simulink model "AdmittanceScanPRBS"  (R2025a)
settings: Solver=VariableStepAuto  StartTime=0.0  StopTime=Tsim  RelTol=1e-3
PreLoadFcn:
  | SimulationTime = 10;
  | AdmittanceScanParameters;
undefined symbols (not defined in the file): Array, Base, BatteryInverter, DiscIntNeverNeededParam, ee_sli_rtmsupport, feeder, fRT, frt, gcbh, GFLBatteryController, GFMBatteryController, gGFM, grid, Grid, line, loadpq, loadstep1, loadstep2, lvrt, LVRT, mGFM, Panel, pll, pmsm, PVController, PVInverter, PVTransformer, scan, time, Ts, VSMbase, windController, windTurbine
libraries: ee_lib x19, eeGeneralControl x17, nesl_utility x16, fl_lib x10, eeTransforms x9, simulink x8, slpidlib x2, batteryecm_lib x1, simulink_extras x1, eePowerMeasurement x1
(part 2 of 4)

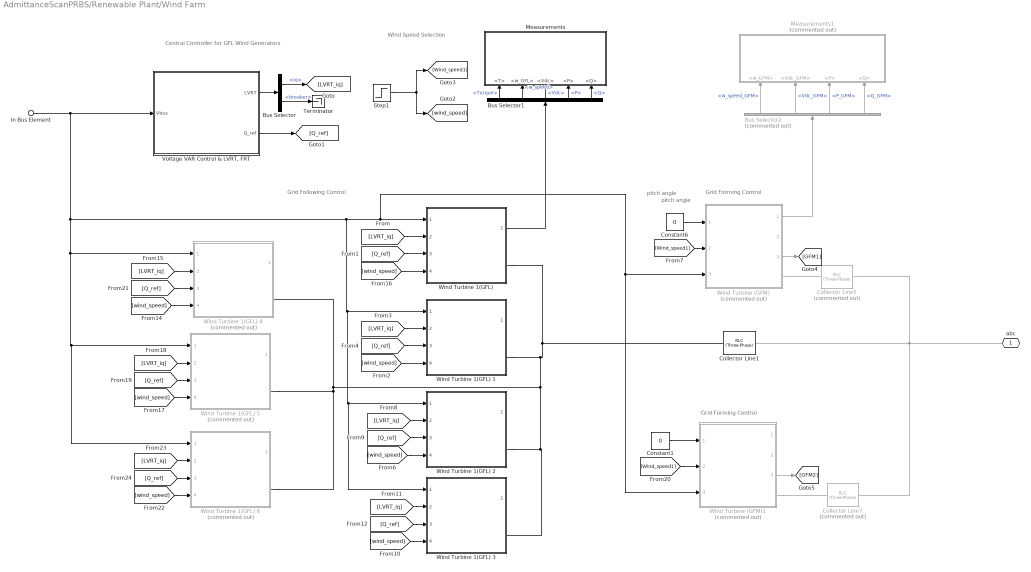
== system AdmittanceScanPRBS/Renewable Plant/Wind Farm ==
  note: Central Controller for GFL Wind Generators
  note: Wind Speed Selection
  note: pitch angle
  note: Grid Following Control
  note: Grid Forming Control
  note: Grid Forming Control
  note: pitch angle
  In Bus Element : Inport  PortName=Vbus
  Bus Selector : BusSelector  OutputSignals=iq,breaker
  Bus Selector1 : BusSelector  OutputSignals=Torque,w_speed,Vdc,P,Q
  Bus Selector2 : BusSelector  Commented=on  OutputSignals=w_speed_GFM,Vdc_GFM,P_GFM,Q_GFM
  Collector Line1 : ee_lib/Passive/RLC Assemblies/RLC (Three-Phase)  port_option=ee.enum.threePhasePort.composite  component_structure=ee.enum.rlc.structure.SeriesRL  R=feeder.r*0.002 Ohm  L=feeder.l*0.002 H  C=1e-6 F  R_parasitic=0 Ohm  G_parasitic=0 1/Ohm  IL_specify=off  IL_priority=High  IL=[0, 0, 0] A  IL_nominal_specify=off  IL_nominal_value=1  IL_nominal_unit=A  VC_specify=off  VC_priority=High  VC=[0, 0, 0] V  VC_nominal_specify=off  VC_nominal_value=1  VC_nominal_unit=V
      settings: InternalSimscapePortConfiguration="{\"Bottom\":[],\"Left\":[{\"id\":\"N1\",\"label\":\"~1\",\"type\":\"foundation.electrical.three_phase\"}],\"Right\":[{\"id\":\"N2\",\"label\":\"~2\",\"type\":\"foundation.electrical.three_phase\"}],\"Top\":[]}"
  Collector Line5 : ee_lib/Passive/RLC Assemblies/RLC (Three-Phase)  Commented=on  port_option=ee.enum.threePhasePort.composite  component_structure=ee.enum.rlc.structure.SeriesRL  R=feeder.r*0.005 Ohm  L=feeder.l*0.005 H  C=1e-6 F  R_parasitic=0 Ohm  G_parasitic=0 1/Ohm  IL_specify=off  IL_priority=High  IL=[0, 0, 0] A  IL_nominal_specify=off  IL_nominal_value=1  IL_nominal_unit=A  VC_specify=off  VC_priority=High  VC=[0, 0, 0] V  VC_nominal_specify=off  VC_nominal_value=1  VC_nominal_unit=V
      settings: InternalSimscapePortConfiguration="{\"Bottom\":[],\"Left\":[{\"id\":\"N1\",\"label\":\"~1\",\"type\":\"foundation.electrical.three_phase\"}],\"Right\":[{\"id\":\"N2\",\"label\":\"~2\",\"type\":\"foundation.electrical.three_phase\"}],\"Top\":[]}"
  Collector Line7 : ee_lib/Passive/RLC Assemblies/RLC (Three-Phase)  Commented=on  port_option=ee.enum.threePhasePort.composite  component_structure=ee.enum.rlc.structure.SeriesRL  R=feeder.r*0.001 Ohm  L=feeder.l*0.001 H  C=1e-6 F  R_parasitic=0 Ohm  G_parasitic=0 1/Ohm  IL_specify=off  IL_priority=High  IL=[0, 0, 0] A  IL_nominal_specify=off  IL_nominal_value=1  IL_nominal_unit=A  VC_specify=off  VC_priority=High  VC=[0, 0, 0] V  VC_nominal_specify=off  VC_nominal_value=1  VC_nominal_unit=V
      settings: InternalSimscapePortConfiguration="{\"Bottom\":[],\"Left\":[{\"id\":\"N1\",\"label\":\"~1\",\"type\":\"foundation.electrical.three_phase\"}],\"Right\":[{\"id\":\"N2\",\"label\":\"~2\",\"type\":\"foundation.electrical.three_phase\"}],\"Top\":[]}"
  Constant1 : Constant  Value=0
  Constant6 : Constant  Value=0
  Measurements : Subsystem
  Measurements1 : Subsystem  Commented=on
  Step1 : Step  Time=time.renewablevariation  Before=12  After=10.5  SampleTime=Ts  ZeroCross=off
  Terminator : Terminator
  "Voltage VAR Control & LVRT, FRT" : Subsystem
      mask Display: image('$imagefile'); % Use "Edit Image" on toolstrip to change.
  Wind Turbine (GFM) : Subsystem  Commented=on  ReferencedSubsystem=gfmWind  Control=VSM Using Turbine Inertia  V_ref=gGFM.vref  Q_ref=gGFM.qref  Kq=gGFM.kq  Kt=gGFM.kt  KqI=mGFM.kq  Kp=mGFM.kp  Kd=gGFM.kd  Kj=gGFM.kj  H=mGFM.h  D=mGFM.d  Vd_ref=mGFM.Vd  frequency1=gGFM.fref  frequency=mGFM.fref  x_vir=mGFM.x_vir  x_vir1=gGFM.r_vir  r_vir1=gGFM.x_vir  Imax1=gGFM.Imax  Imax=mGFM.Imax  r_vir=mGFM.r_vir  Kpq_mpp=pmsm.lq*pmsm.alpha  Kpd_mpp=pmsm.ld*pmsm.alpha  Kiq_mpp=pmsm.rs*pmsm.alpha  Kid_mpp=pmsm.rs*pmsm.alpha  Kpq=pmsm.lq*pmsm.alpha  Kpd=pmsm.ld*pmsm.alpha  Kiq=pmsm.rs*pmsm.alpha  Kid=pmsm.rs*pmsm.alpha  Kp_dc_sm=mGFM.kpdc  Ki_dc_sm=mGFM.kidc  wt1=0.01  rt1=0.01  pitch1=windTurbine.pitch  cp1=windTurbine.cp  airDensity1=windTurbine.airDensity  TSR1=windTurbine.TSR  Radius1=windTurbine.turbineRadius  wt=0.01  rt=0.01  pitch=windTurbine.pitch  cp=windTurbine.cp  airDensity=windTurbine.airDensity  Radius=windTurbine.turbineRadius  TSR=windTurbine.TSR  Inertia1=windTurbine.inertia  Inertia=windTurbine.inertia  psim1=pmsm.psim  p1=pmsm.p  Rs1=pmsm.rs  Lq1=pmsm.lq  Ld1=pmsm.ld  Ld=pmsm.ld  Lq=pmsm.lq  Rs=pmsm.rs  p=pmsm.p  psim=pmsm.psim
  Wind Turbine (GFM)1 : Subsystem  Commented=on  ReferencedSubsystem=gfmWind  Control=VSM Using Turbine Inertia  V_ref=gGFM.vref  Q_ref=gGFM.qref  Kq=gGFM.kq  Kt=gGFM.kt  KqI=mGFM.kq  Kp=mGFM.kp  Kd=gGFM.kd  Kj=gGFM.kj  H=mGFM.h  D=mGFM.d  Vd_ref=mGFM.Vd  frequency1=gGFM.fref  frequency=mGFM.fref  x_vir=mGFM.x_vir  x_vir1=gGFM.r_vir  r_vir1=gGFM.x_vir  Imax1=gGFM.Imax  Imax=mGFM.Imax  r_vir=mGFM.r_vir  Kpq_mpp=pmsm.lq*pmsm.alpha  Kpd_mpp=pmsm.ld*pmsm.alpha  Kiq_mpp=pmsm.rs*pmsm.alpha  Kid_mpp=pmsm.rs*pmsm.alpha  Kpq=pmsm.lq*pmsm.alpha  Kpd=pmsm.ld*pmsm.alpha  Kiq=pmsm.rs*pmsm.alpha  Kid=pmsm.rs*pmsm.alpha  Kp_dc_sm=mGFM.kpdc  Ki_dc_sm=mGFM.kidc  wt1=0.01  rt1=0.01  pitch1=windTurbine.pitch  cp1=windTurbine.cp  airDensity1=windTurbine.airDensity  TSR1=windTurbine.TSR  Radius1=windTurbine.turbineRadius  wt=0.01  rt=0.01  pitch=windTurbine.pitch  cp=windTurbine.cp  airDensity=windTurbine.airDensity  Radius=windTurbine.turbineRadius  TSR=windTurbine.TSR  Inertia1=windTurbine.inertia  Inertia=windTurbine.inertia  psim1=pmsm.psim  p1=pmsm.p  Rs1=pmsm.rs  Lq1=pmsm.lq  Ld1=pmsm.ld  Ld=pmsm.ld  Lq=pmsm.lq  Rs=pmsm.rs  p=pmsm.p  psim=pmsm.psim
  Wind Turbine 1(GFL) : Subsystem  ReferencedSubsystem=WindGFLMpp  p=pmsm.p  psim=pmsm.psim  Rs=pmsm.rs  Ld=pmsm.ld  Lq=pmsm.lq  Kdip_sm=pmsm.ld*pmsm.alpha  Kdii_sm=pmsm.rs*pmsm.alpha  Kqip_sm=pmsm.lq*pmsm.alpha  Kqii_sm=pmsm.rs*pmsm.alpha  airDensity=windTurbine.airDensity  turbineRadius=windTurbine.turbineRadius  pitch=windTurbine.pitch  TSR=windTurbine.TSR  cp=windTurbine.cp  wt=0.01  rt=0.01  Inertia=windTurbine.inertia  Kp_dc=windController.kpv  Ki_dc=windController.kiv  Kdpi_g=windController.kpic  Kdii_g=windController.kiic  Kqpi_g=windController.kpic  Kqii_g=windController.kiic
  Wind Turbine 1(GFL) 1 : Subsystem  ReferencedSubsystem=WindGFLMpp  p=pmsm.p  psim=pmsm.psim  Rs=pmsm.rs  Ld=pmsm.ld  Lq=pmsm.lq  Kdip_sm=pmsm.ld*pmsm.alpha  Kdii_sm=pmsm.rs*pmsm.alpha  Kqip_sm=pmsm.lq*pmsm.alpha  Kqii_sm=pmsm.rs*pmsm.alpha  airDensity=windTurbine.airDensity  turbineRadius=windTurbine.turbineRadius  pitch=windTurbine.pitch  TSR=windTurbine.TSR  cp=windTurbine.cp  wt=0.01  rt=0.01  Inertia=windTurbine.inertia  Kp_dc=windController.kpv  Ki_dc=windController.kiv  Kdpi_g=windController.kpic  Kdii_g=windController.kiic  Kqpi_g=windController.kpic  Kqii_g=windController.kiic
  Wind Turbine 1(GFL) 2 : Subsystem  ReferencedSubsystem=WindGFLMpp  p=pmsm.p  psim=pmsm.psim  Rs=pmsm.rs  Ld=pmsm.ld  Lq=pmsm.lq  Kdip_sm=pmsm.ld*pmsm.alpha  Kdii_sm=pmsm.rs*pmsm.alpha  Kqip_sm=pmsm.lq*pmsm.alpha  Kqii_sm=pmsm.rs*pmsm.alpha  airDensity=windTurbine.airDensity  turbineRadius=windTurbine.turbineRadius  pitch=windTurbine.pitch  TSR=windTurbine.TSR  cp=windTurbine.cp  wt=0.01  rt=0.01  Inertia=windTurbine.inertia  Kp_dc=windController.kpv  Ki_dc=windController.kiv  Kdpi_g=windController.kpic  Kdii_g=windController.kiic  Kqpi_g=windController.kpic  Kqii_g=windController.kiic
  Wind Turbine 1(GFL) 3 : Subsystem  ReferencedSubsystem=WindGFLMpp  p=pmsm.p  psim=pmsm.psim  Rs=pmsm.rs  Ld=pmsm.ld  Lq=pmsm.lq  Kdip_sm=pmsm.ld*pmsm.alpha  Kdii_sm=pmsm.rs*pmsm.alpha  Kqip_sm=pmsm.lq*pmsm.alpha  Kqii_sm=pmsm.rs*pmsm.alpha  airDensity=windTurbine.airDensity  turbineRadius=windTurbine.turbineRadius  pitch=windTurbine.pitch  TSR=windTurbine.TSR  cp=windTurbine.cp  wt=0.01  rt=0.01  Inertia=windTurbine.inertia  Kp_dc=windController.kpv  Ki_dc=windController.kiv  Kdpi_g=windController.kpic  Kdii_g=windController.kiic  Kqpi_g=windController.kpic  Kqii_g=windController.kiic
  Wind Turbine 1(GFL) 4 : Subsystem  Commented=on  ReferencedSubsystem=WindGFLMpp  p=pmsm.p  psim=pmsm.psim  Rs=pmsm.rs  Ld=pmsm.ld  Lq=pmsm.lq  Kdip_sm=pmsm.ld*pmsm.alpha  Kdii_sm=pmsm.rs*pmsm.alpha  Kqip_sm=pmsm.lq*pmsm.alpha  Kqii_sm=pmsm.rs*pmsm.alpha  airDensity=windTurbine.airDensity  turbineRadius=windTurbine.turbineRadius  pitch=windTurbine.pitch  TSR=windTurbine.TSR  cp=windTurbine.cp  wt=0.01  rt=0.01  Inertia=windTurbine.inertia  Kp_dc=windController.kpv  Ki_dc=windController.kiv  Kdpi_g=windController.kpic  Kdii_g=windController.kiic  Kqpi_g=windController.kpic  Kqii_g=windController.kiic
  Wind Turbine 1(GFL) 5 : Subsystem  Commented=on  ReferencedSubsystem=WindGFLMpp  p=pmsm.p  psim=pmsm.psim  Rs=pmsm.rs  Ld=pmsm.ld  Lq=pmsm.lq  Kdip_sm=pmsm.ld*pmsm.alpha  Kdii_sm=pmsm.rs*pmsm.alpha  Kqip_sm=pmsm.lq*pmsm.alpha  Kqii_sm=pmsm.rs*pmsm.alpha  airDensity=windTurbine.airDensity  turbineRadius=windTurbine.turbineRadius  pitch=windTurbine.pitch  TSR=windTurbine.TSR  cp=windTurbine.cp  wt=0.01  rt=0.01  Inertia=windTurbine.inertia  Kp_dc=windController.kpv  Ki_dc=windController.kiv  Kdpi_g=windController.kpic  Kdii_g=windController.kiic  Kqpi_g=windController.kpic  Kqii_g=windController.kiic
  Wind Turbine 1(GFL) 6 : Subsystem  Commented=on  ReferencedSubsystem=WindGFLMpp  p=pmsm.p  psim=pmsm.psim  Rs=pmsm.rs  Ld=pmsm.ld  Lq=pmsm.lq  Kdip_sm=pmsm.ld*pmsm.alpha  Kdii_sm=pmsm.rs*pmsm.alpha  Kqip_sm=pmsm.lq*pmsm.alpha  Kqii_sm=pmsm.rs*pmsm.alpha  airDensity=windTurbine.airDensity  turbineRadius=windTurbine.turbineRadius  pitch=windTurbine.pitch  TSR=windTurbine.TSR  cp=windTurbine.cp  wt=0.01  rt=0.01  Inertia=windTurbine.inertia  Kp_dc=windController.kpv  Ki_dc=windController.kiv  Kdpi_g=windController.kpic  Kdii_g=windController.kiic  Kqpi_g=windController.kpic  Kqii_g=windController.kiic
  abc : PMIOPort  Side=Right
  wires:
  "Voltage VAR Control & LVRT, FRT"/1(LVRT) -> Bus Selector/1
  Bus Selector/2 -> Terminator/1  "<breaker>"
  Bus Selector1/4 -> Measurements/4(<P>)  "<P>"
  Bus Selector1/5 -> Measurements/5(<Q>)  "<Q>"
  Bus Selector1/1 -> Measurements/1(<T>)  "<Torque>"
  Bus Selector1/3 -> Measurements/3(<Vdc>)  "<Vdc>"
  Bus Selector1/2 -> Measurements/2(<w_GFL>)  "<w_speed>"
  "Voltage VAR Control & LVRT, FRT"/2(Q_ref) -> [Q_ref]
  Bus Selector/1 -> [LVRT_iq]  "<iq>"
  Wind Turbine 1(GFL)/1 -> Bus Selector1/1
  Wind Turbine (GFM)/3 -> [GFM1]
  Bus Selector2/4 -> Measurements1/4(<Q>)  "<Q_GFM>"
  Bus Selector2/3 -> Measurements1/3(<P>)  "<P_GFM>"
  Bus Selector2/1 -> Measurements1/1(<w_GFM>)  "<w_speed_GFM>"
  Bus Selector2/2 -> Measurements1/2(<Vdc_GFM>)  "<Vdc_GFM>"
  Wind Turbine (GFM)/1 -> Bus Selector2/1
  Step1/1 -> [Wind_speed1], [wind_speed]
  [LVRT_iq] -> Wind Turbine 1(GFL) 4/2
  [Q_ref] -> Wind Turbine 1(GFL) 4/3
  [wind_speed] -> Wind Turbine 1(GFL) 4/4
  [LVRT_iq] -> Wind Turbine 1(GFL) 5/2
  [Q_ref] -> Wind Turbine 1(GFL) 5/3
  [wind_speed] -> Wind Turbine 1(GFL) 5/4
  [LVRT_iq] -> Wind Turbine 1(GFL) 6/2
  [Q_ref] -> Wind Turbine 1(GFL) 6/3
  [wind_speed] -> Wind Turbine 1(GFL) 6/4
  [LVRT_iq] -> Wind Turbine 1(GFL)/2
  [Q_ref] -> Wind Turbine 1(GFL)/3
  [wind_speed] -> Wind Turbine 1(GFL)/4
  [LVRT_iq] -> Wind Turbine 1(GFL) 1/2
  [Q_ref] -> Wind Turbine 1(GFL) 1/3
  [wind_speed] -> Wind Turbine 1(GFL) 1/4
  [LVRT_iq] -> Wind Turbine 1(GFL) 2/2
  [Q_ref] -> Wind Turbine 1(GFL) 2/3
  [wind_speed] -> Wind Turbine 1(GFL) 2/4
  [LVRT_iq] -> Wind Turbine 1(GFL) 3/2
  [Q_ref] -> Wind Turbine 1(GFL) 3/3
  [wind_speed] -> Wind Turbine 1(GFL) 3/4
  Constant6/1 -> Wind Turbine (GFM)/1
  [Wind_speed1] -> Wind Turbine (GFM)/2
  Constant1/1 -> Wind Turbine (GFM)1/1
  [Wind_speed1] -> Wind Turbine (GFM)1/2
  Wind Turbine (GFM)1/3 -> [GFM2]
  In Bus Element/1 -> Wind Turbine 1(GFL) 3/1, Wind Turbine 1(GFL) 2/1, Wind Turbine 1(GFL) 1/1, Wind Turbine (GFM)1/3, Wind Turbine (GFM)/3, Wind Turbine 1(GFL)/1, Wind Turbine 1(GFL) 6/1, Wind Turbine 1(GFL) 5/1, Wind Turbine 1(GFL) 4/1, "Voltage VAR Control & LVRT, FRT"/1(Vbus)
  connections:
  Wind Turbine (GFM)/RConn1 -- Collector Line5/LConn1
  Wind Turbine (GFM)1/RConn1 -- Collector Line7/LConn1
  Wind Turbine 1(GFL) 4/RConn1 -- Wind Turbine 1(GFL) 6/RConn1 -- Wind Turbine 1(GFL) 5/RConn1 -- Wind Turbine 1(GFL) 3/RConn1 -- Wind Turbine 1(GFL) 2/RConn1 -- Wind Turbine 1(GFL) 1/RConn1 -- Collector Line1/LConn1 -- Wind Turbine 1(GFL)/RConn1
  Collector Line7/RConn1 -- Collector Line1/RConn1 -- Collector Line5/RConn1 -- abc/RConn1

== system AdmittanceScanPRBS/PLL & Measurements/PLL/Sinusoidal Measurement (PLL, Three-Phase)1 ==
  note: Loop Filter (LF)
  note: Voltage-controlled oscillator (VCO)
  abc : Inport  PortDimensions=3  SampleTime=Ts
  Angle : Subsystem
  Low-Pass Filter (Discrete or Continuous) : eeGeneralControl/Low-Pass Filter (Discrete or Continuous)  K=1/2/pi  T=1e-3  B=inf  A=-inf  init_option=Specify as parameter  x0=F0  Ts=Ts
      settings: LibrarySourceBlock=|
      | eeSinusoidalMeasurementV2/Sinusoidal Measurement
      | (PLL, Three-Phase)/Low-Pass Filter
      | (Discrete or Continuous)
  Moving Average (Variable Frequency) : eeGeneralControl/Moving Average (Variable Frequency)  VariantControl=Variant1  LabelModeActiveChoice=Discrete  f0=F0  fmin=5  x0=0  BufferSize=8192  Ts=Ts
      settings: LibrarySourceBlock=|
      | eeSinusoidalMeasurementV2/Sinusoidal Measurement
      | (PLL, Three-Phase)/Moving Average
      | (Variable Frequency)
  PI : Subsystem
  Park Transform : eeTransforms/Park Transform  AxisAlignment=Q-axis  PowerInvariant=off
  Pythagorian Sum : Fcn  Expr=sqrt(u(1)^2+u(2)^2)
  Selector2 : Selector  InputPortWidth=3  IndexOptions=Index vector (dialog)  Indices=[2]  OutputSizes=1
  freq : Outport  VectorParamsAs1DForOutWhenUnconnected=off
  angle : Outport  Port=2  VectorParamsAs1DForOutWhenUnconnected=off
  mag : Outport  Port=3  VectorParamsAs1DForOutWhenUnconnected=off
  wires:
  Moving Average (Variable Frequency)/1 -> Selector2/1, Pythagorian Sum/1
  Selector2/1 -> PI/1(u)
  Low-Pass Filter (Discrete or Continuous)/1 -> freq/1, Moving Average (Variable Frequency)/1
  Angle/1(theta) -> angle/1, Park Transform/2
  PI/1(y) -> Angle/1(omega), Low-Pass Filter (Discrete or Continuous)/1
  Park Transform/1 -> Moving Average (Variable Frequency)/2
  Pythagorian Sum/1 -> mag/1
  abc/1 -> Park Transform/1

== system AdmittanceScanPRBS/Renewable Plant/PV Plant/100 MWp PV Park ==
  note: PV Park
  LVRT_iq : Inport
  Q_ref : Inport  Port=2
  "Current and Voltage Sensor " : ee_lib/Sensors & Transducers/Current and Voltage Sensor (Three-Phase)  vMeasurementType=ee.enum.vmeasurement.lg  outputUnit=ee.enum.unit.pu  SRated=Base.MVA_base_new A*V  VRated=Base.KV_base_new V  I_specify=off  I_priority=None  I=[0, 0, 0] A  I_nominal_specify=off  I_nominal_value=1  I_nominal_unit=A  V_specify=off  V_priority=None  V=[0, 0, 0] V  V_nominal_specify=off  V_nominal_value=1  V_nominal_unit=V
      settings: InternalSimscapePortConfiguration="{\"Bottom\":[],\"Left\":[{\"id\":\"N1\",\"label\":\"~1\",\"type\":\"foundation.electrical.three_phase\"}],\"Right\":[{\"id\":\"V_output\",\"label\":\"V\",\"type\":\"output\"},{\"id\":\"I_output\",\"label\":\"I\",\"type\":\"output\"},{\"id\":\"N2\",\"label\":\"~2\",\"type\":\"foundation.electrical.three_phase\"}],\"Top\":[]}"
  PS-Simulink Converter25 : nesl_utility/PS-Simulink Converter  PhysicalDomain=network_engine_domain  SubClassName=ps_output  LeftPortType=input  RightPortType=output  PseudoPeriodic=off  Frequencies=[]  VectorFormat=inherit  Unit=inherit  AffineConversion=off
  PV Inverter A2 : Subsystem
  Step2 : Step  Time=time.renewablevariation  Before=600  After=650  SampleTime=Ts
  PV : PMIOPort  Side=Left
  IPV : Outport
  wires:
  PS-Simulink Converter25/1 -> IPV/1
  Q_ref/1 -> PV Inverter A2/3(Q_ref)
  Step2/1 -> PV Inverter A2/1(Insolation1)
  LVRT_iq/1 -> PV Inverter A2/2(LVRT)
  connections:
  PV/RConn1 -- "Current and Voltage Sensor "/RConn3
  PS-Simulink Converter25/LConn1 -- "Current and Voltage Sensor "/RConn2
  PV Inverter A2/RConn1 -- "Current and Voltage Sensor "/LConn1

== system AdmittanceScanPRBS/Renewable Plant/PV Plant/60 MWhr Battery Energy Storage ==
  In Bus Element : Inport  PortName=Vbus
  LVRT_iq : Inport  Port=2
  Current and Voltage Sensor (Three-Phase)5 : ee_lib/Sensors & Transducers/Current and Voltage Sensor (Three-Phase)  vMeasurementType=ee.enum.vmeasurement.lg  outputUnit=ee.enum.unit.pu  SRated=Base.MVA_base_new A*V  VRated=Base.KV_base_new V  I_specify=off  I_priority=None  I=[0, 0, 0] A  I_nominal_specify=off  I_nominal_value=1  I_nominal_unit=A  V_specify=off  V_priority=None  V=[0, 0, 0] V  V_nominal_specify=off  V_nominal_value=1  V_nominal_unit=V
      settings: InternalSimscapePortConfiguration="{\"Bottom\":[],\"Left\":[{\"id\":\"N1\",\"label\":\"~1\",\"type\":\"foundation.electrical.three_phase\"}],\"Right\":[{\"id\":\"V_output\",\"label\":\"V\",\"type\":\"output\"},{\"id\":\"I_output\",\"label\":\"I\",\"type\":\"output\"},{\"id\":\"N2\",\"label\":\"~2\",\"type\":\"foundation.electrical.three_phase\"}],\"Top\":[]}"
  Inverter and DC-DC Converter : Subsystem
  L Filter : ee_lib/Passive/RLC Assemblies/RLC (Three-Phase)  port_option=ee.enum.threePhasePort.composite  component_structure=ee.enum.rlc.structure.L  R=1e-3 Ohm  L=PVInverter.L H  C=1e-6 F  R_parasitic=0 Ohm  G_parasitic=0 1/Ohm  IL_specify=off  IL_priority=High  IL=[0, 0, 0] A  IL_nominal_specify=off  IL_nominal_value=1  IL_nominal_unit=A  VC_specify=off  VC_priority=High  VC=[0, 0, 0] V  VC_nominal_specify=off  VC_nominal_value=1  VC_nominal_unit=V
      settings: InternalSimscapePortConfiguration="{\"Bottom\":[],\"Left\":[{\"id\":\"N1\",\"label\":\"~1\",\"type\":\"foundation.electrical.three_phase\"}],\"Right\":[{\"id\":\"N2\",\"label\":\"~2\",\"type\":\"foundation.electrical.three_phase\"}],\"Top\":[]}"
  Measurement5 : Subsystem
  PS-Simulink Converter10 : nesl_utility/PS-Simulink Converter  PhysicalDomain=network_engine_domain  SubClassName=ps_output  LeftPortType=input  RightPortType=output  PseudoPeriodic=off  Frequencies=[]  VectorFormat=inherit  Unit=inherit  AffineConversion=off
  PS-Simulink Converter9 : nesl_utility/PS-Simulink Converter  PhysicalDomain=network_engine_domain  SubClassName=ps_output  LeftPortType=input  RightPortType=output  PseudoPeriodic=off  Frequencies=[]  VectorFormat=inherit  Unit=inherit  AffineConversion=off
  Variant Subsystem : Subsystem  Variant=on  VariantControlMode=label  LabelModeActiveChoice=BESSGridSupporting  mask{LabelModeActiveChoice=BESSGridSupporting}
      mask prompts: LabelModeActiveChoice "Choose BESS Controller"
      mask TypeOptions LabelModeActiveChoice: LabelModeActiveChoice
  abc : PMIOPort  Side=Right
  Bat : Outport
  wires:
  In Bus Element/1 -> Variant Subsystem/2(Vbus)
  Variant Subsystem/1(mabc) -> Inverter and DC-DC Converter/1(m_abc)
  PS-Simulink Converter9/1 -> Measurement5/2(u)
  PS-Simulink Converter10/1 -> Measurement5/1(In1)
  Measurement5/2(Bat) -> Bat/1, Variant Subsystem/4(Bat)
  LVRT_iq/1 -> Variant Subsystem/3(LVRT_iq)
  Measurement5/1(ipv1) -> Variant Subsystem/1(ipv2)
  connections:
  abc/RConn1 -- Current and Voltage Sensor (Three-Phase)5/RConn3
  Inverter and DC-DC Converter/RConn1 -- L Filter/LConn1
  Current and Voltage Sensor (Three-Phase)5/LConn1 -- L Filter/RConn1
  Current and Voltage Sensor (Three-Phase)5/RConn1 -- PS-Simulink Converter10/LConn1
  PS-Simulink Converter9/LConn1 -- Current and Voltage Sensor (Three-Phase)5/RConn2

== system AdmittanceScanPRBS/Renewable Plant/PV Plant/PV Plant Controller  ==
  In Bus Element14 : Inport  PortName=Vbus
  Terminator : Terminator
  "Voltage VAR Control & LVRT, FRT" : Subsystem
      mask Display: image('$imagefile'); % Use "Edit Image" on toolstrip to change.
  Q_ref : Outport
  wires:
  In Bus Element14/1 -> "Voltage VAR Control & LVRT, FRT"/1(Vbus)
  "Voltage VAR Control & LVRT, FRT"/2(Q_ref) -> Q_ref/1
  "Voltage VAR Control & LVRT, FRT"/1(LVRT) -> Terminator/1

== system AdmittanceScanPRBS/Renewable Plant/Wind Farm/Measurements ==
  <T> : Inport
  <w_GFL> : Inport  Port=2
  <Vdc> : Inport  Port=3
  <P> : Inport  Port=4
  <Q> : Inport  Port=5
  Terminator{,1..4} (5 alike) : Terminator
  wires:
  <Vdc>/1 -> Terminator2/1  "Vdc_GFL"
  <Q>/1 -> Terminator4/1
  <w_GFL>/1 -> Terminator1/1
  <T>/1 -> Terminator/1
  <P>/1 -> Terminator3/1

== system AdmittanceScanPRBS/Renewable Plant/Wind Farm/Measurements1 ==
  <w_GFM> : Inport
  <Vdc_GFM> : Inport  Port=2
  <P> : Inport  Port=3
  <Q> : Inport  Port=4
  Terminator{1..4} (4 alike) : Terminator
  wires:
  <P>/1 -> Terminator3/1
  <w_GFM>/1 -> Terminator1/1
  <Q>/1 -> Terminator4/1
  <Vdc_GFM>/1 -> Terminator2/1

== system AdmittanceScanPRBS/Renewable Plant/Wind Farm/Voltage VAR Control & LVRT, FRT ==
  In Bus Element : Inport  PortName=Vbus  Element=Vmag
  In Bus Element1 : Inport  PortName=Vbus  Element=w
  Data Type Conversion : DataTypeConversion  RndMeth=Nearest  SaturateOnIntegerOverflow=off
  Delay : Delay  DelayLength=100
  Frequency RideThrough : Subsystem
  LVRT Characterstics : Subsystem
  OR : Logic  Operator=OR  IconShape=distinctive  AllPortsSameDT=off  OutDataTypeStr=boolean
  Unit Delay : UnitDelay  SampleTime=-1  HasFrameUpgradeWarning=on
  V_ref : Constant  Value=windController.vRef  SampleTime=Ts
  Voltage Control : Subsystem
  Out Bus Element : Outport  PortName=LVRT  Element=breaker
  Out Bus Element1 : Outport  PortName=LVRT  Element=iq
  Q_ref : Outport  Port=2
  wires:
  In Bus Element/1 -> LVRT Characterstics/1(Vmag), Voltage Control/1(In1)
  LVRT Characterstics/2(iq) -> Out Bus Element1/1
  V_ref/1 -> Voltage Control/2(In2)
  Voltage Control/1(Out1) -> Delay/1
  OR/1 -> Data Type Conversion/1
  LVRT Characterstics/1(Trip Signal) -> OR/1
  In Bus Element1/1 -> Frequency RideThrough/1(f)
  Data Type Conversion/1 -> Unit Delay/1
  Frequency RideThrough/1(Trip  Signal) -> OR/2
  Unit Delay/1 -> Out Bus Element/1
  Delay/1 -> Q_ref/1

== system AdmittanceScanPRBS/PLL & Measurements/PLL/Sinusoidal Measurement (PLL, Three-Phase)1/Angle ==
  omega : Inport
  Integrator with Wrapped State (Discrete or Continuous) : eeGeneralControl/Integrator with Wrapped State (Discrete or Continuous)  LabelModeActiveChoice=Discrete  WrappedStateUpperValue=2*pi  WrappedStateLowerValue=0  x0=Theta0  Ts=Ts
      settings: LibrarySourceBlock=|
      | eeSinusoidalMeasurementV2/Sinusoidal Measurement
      | (PLL, Three-Phase)/Angle/Integrator with
      | Wrapped State
      | (Discrete or Continuous)
  theta : Outport  VectorParamsAs1DForOutWhenUnconnected=off
  wires:
  Integrator with Wrapped State (Discrete or Continuous)/1 -> theta/1
  omega/1 -> Integrator with Wrapped State (Discrete or Continuous)/1

== system AdmittanceScanPRBS/PLL & Measurements/PLL/Sinusoidal Measurement (PLL, Three-Phase)1/PI ==
  u : Inport
  Constant : Constant  Value=2*pi*F0  SampleTime=Ts
  Constant1 : Constant  Value=0  SampleTime=Ts
  Data Type Conversion Inherited : simulink/Signal Attributes/Data Type Conversion Inherited  ConvertRealWorld=Real World Value  DoSatur=off
  Gain : Gain  Gain=Kp_LF
  Gain1 : Gain  Gain=Ki_LF
  Integrator (Discrete or Continuous) : eeGeneralControl/Integrator (Discrete or Continuous)  LabelModeActiveChoice=Discrete  IntegratorMethod=Integration: Forward Euler  ExternalReset=level  LimitType=Anti-windup  B=inf  A=-inf  Ts=Ts
      settings: LibrarySourceBlock=|
      | eeSinusoidalMeasurementV2/Sinusoidal Measurement
      | (PLL, Three-Phase)/PI/Integrator
      | (Discrete or Continuous)
  Sum : Sum  Inputs=|++
  y : Outport  VectorParamsAs1DForOutWhenUnconnected=off
  wires:
  Constant/1 -> Data Type Conversion Inherited/2
  Data Type Conversion Inherited/1 -> Integrator (Discrete or Continuous)/3
  Gain1/1 -> Integrator (Discrete or Continuous)/1
  u/1 -> Gain1/1, Data Type Conversion Inherited/1, Gain/1
  Gain/1 -> Sum/1
  Integrator (Discrete or Continuous)/1 -> Sum/2
  Sum/1 -> y/1
  Constant1/1 -> Integrator (Discrete or Continuous)/2

== system AdmittanceScanPRBS/Renewable Plant/PV Plant/100 MWp PV Park/PV Inverter A2 ==
  Insolation1 : Inport
  In Bus Element3 : Inport  Port=2  PortName=LVRT
  Q_ref : Inport  Port=3
  PV Array : ee_lib/Sources/Solar Cell  prm=3  Isc=3.8 A  Voc=0.586 V  Is=SolarCell.diode_saturation_current A  Is2=0 A  Iph=SolarCell.solar_generated_current_AM A  Ir0=1000 W/m^2  ec=SolarCell.quality_factor_i  N2=SolarCell.quality_factor_j  Rs=SolarCell.series_resistance Ohm  Rp=SolarCell.parallel_resistance Ohm  N_series=Panel.n_series_cell_panel*Array.n_series_panels_per_string  N_parallel=Panel.n_parallel_strings_panel*Array.n_parallel_strings  TIPH1=SolarCell.temp_cofficient 1/K  EG=SolarCell.Eg eV  TXIS1=SolarCell.temperature_exponent_Is1  TXIS2=SolarCell.temperature_exponent_Is2  TRS1=SolarCell.temperature_exponent_Rs  TRP1=SolarCell.temperature_exponent_Rp  Tmeas=SolarCell.measurement_temperature degC  TFIXED=SolarCell.device_temperature degC  thermal_mass=100 J/K  initial_temperature=25 degC
  Simulink-PS Converter1 : nesl_utility/Simulink-PS Converter  PhysicalDomain=network_engine_domain  SubClassName=ps_input  LeftPortType=input  RightPortType=output  PseudoPeriodic=off  Frequencies=[]  NoiseDistribution=none  NoiseParameters=[]  Unit=1  AffineConversion=off  FilteringAndDerivatives=provide  SimscapeFilterOrder=1  InputFilterTimeConstant=0.001  UdotUserProvided=0
  Simulink-PS Converter2 : nesl_utility/Simulink-PS Converter  PhysicalDomain=network_engine_domain  SubClassName=ps_input  LeftPortType=input  RightPortType=output  PseudoPeriodic=off  Frequencies=[]  NoiseDistribution=none  NoiseParameters=[]  Unit=1  AffineConversion=off  FilteringAndDerivatives=provide  SimscapeFilterOrder=1  InputFilterTimeConstant=0.001  UdotUserProvided=0
  Subsystem Reference : Subsystem  ReferencedSubsystem=PVInverterGFL  c=PVInverter.C F  g=0 1/Ohm  vc_priority=None  vc_specify=on  vc=PVInverter.Vdc V  Pfixed=1 W  L=PVInverter.L H  R=1e-3 Ohm  VRated=Base.KV_base_new  SRated=Base.MVA_base_new
  Subsystem Reference1 : Subsystem  ReferencedSubsystem=PVcontroller  L=PVInverter.L  frequency=Grid.frequency  iMax=PVInverter.I_max_pu  zBase=Base.z_base  mVAbase=Base.MVA_base_new  VdcBase=PVController.Vdc_base  sampleTime=-1  Choice=Incremental conductance (INC)  Vdc=PVInverter.Vdc  delV=3  tSettling=Mpp.ts  Kppll=PLL.Kp_pll  Kipll=PLL.Ki_pll  initialPhase=0  Kpv=PVController.Kp_v  Kiv=PVController.Ki_v  Kdv=0  Kpicd=PVController.Kp_ic  Kiicd=PVController.Ki_ic  Kdicd=0  Kpicq=PVController.Kp_ic  Kiicq=PVController.Ki_ic  Kdicq=0
  Unit Delay2 : UnitDelay  SampleTime=Ts  HasFrameUpgradeWarning=on
  abc : PMIOPort  Side=Right
  wires:
  Unit Delay2/1 -> Simulink-PS Converter2/1
  Q_ref/1 -> Subsystem Reference1/1
  Insolation1/1 -> Simulink-PS Converter1/1
  In Bus Element3/1 -> Subsystem Reference1/6
  Subsystem Reference/1 -> Subsystem Reference1/2
  Subsystem Reference/2 -> Subsystem Reference1/3
  Subsystem Reference/3 -> Subsystem Reference1/4
  Subsystem Reference/4 -> Subsystem Reference1/5
  Subsystem Reference1/1 -> Unit Delay2/1
  connections:
  PV Array/LConn1 -- Simulink-PS Converter1/RConn1
  Subsystem Reference/LConn2 -- PV Array/LConn2
  Subsystem Reference/LConn1 -- Simulink-PS Converter2/RConn1
  Subsystem Reference/LConn3 -- PV Array/RConn1
  abc/RConn1 -- Subsystem Reference/LConn4

== system AdmittanceScanPRBS/Renewable Plant/PV Plant/60 MWhr Battery Energy Storage/Inverter and DC-DC Converter ==
  m_abc : Inport
  Average-Value Voltage Source Converter (Three-Phase) : ee_lib/Semiconductors & Converters/Converters/Average-Value Voltage Source Converter (Three-Phase)  port_option=ee.enum.threePhasePort.composite  frequency_option=ee.enum.converters.frequency.variable  input_option=ee.enum.converters.inputOption.ModWave  FRated=60 Hz  losses_parameterization=ee.enum.converters.losses.fixed  Pfixed=1 W  ks=0.01  kc1=1.7 V  kc2=0.01 Ohm  Ploss_vect=[100, 800, 1870, 3250, 4900] W  Irms_vect=[10, 100, 200, 300, 400] A  Vdc_nom=300 V  thermal_mass=30000 J/K  temperature_specify=off  temperature_priority=High  temperature=298.15 K  temperature_nominal_specify=off  temperature_nominal_value=1  temperature_nominal_unit=K
      settings: InternalSimscapePortConfiguration="{\"Bottom\":[],\"Left\":[{\"id\":\"ModWave\",\"label\":\"ModWave\",\"type\":\"input\"},{\"id\":\"N\",\"label\":\"~\",\"type\":\"foundation.electrical.three_phase\"}],\"Right\":[{\"id\":\"p\",\"label\":\"+\",\"type\":\"foundation.electrical.electrical\"},{\"id\":\"n\",\"label\":\"-\",\"type\":\"foundation.electrical.electrical\"}],\"Top\":[]}"
  Average-Value DC-DC Converter : ee_lib/Semiconductors & Converters/Converters/Average-Value DC-DC Converter  implementation_option=ee.enum.converters.implementation.behavioral  converter_type=ee.enum.converters.dcdctype.buckboost  control_option=ee.enum.converters.controlinput.voltage  efficiency_option=ee.enum.converters.efficiency.constant  efficiency_fixed=99  i_vec=[0, 2, 5] A  efficiency_vec=[90, 95, 98]  Lf=1e-6 H  Rl=0 Ohm  Cf=1e-7 F  Rc=1e-6 Ohm  iL_specify=off  iL_priority=High  iL=0 A  iL_nominal_specify=off  iL_nominal_value=1  iL_nominal_unit=A  vc_specify=off  vc_priority=High  vc=0 V  vc_nominal_specify=off  vc_nominal_value=1  vc_nominal_unit=V
      settings: InternalSimscapePortConfiguration="{\"Bottom\":[],\"Left\":[{\"id\":\"Vref\",\"label\":\"Vref\",\"type\":\"input\"},{\"id\":\"p1\",\"label\":\"1+\",\"type\":\"foundation.electrical.electrical\"},{\"id\":\"n1\",\"label\":\"1-\",\"type\":\"foundation.electrical.electrical\"}],\"Right\":[{\"id\":\"p2\",\"label\":\"2+\",\"type\":\"foundation.electrical.electrical\"},{\"id\":\"n2\",\"label\":\"2-\",\"type\":\"foundation.electrical.electrical\"}],\"Top\":[]}"
  Capacitor : fl_lib/Electrical/Electrical Elements/Capacitor  c=GFMBatteryController.C_dc F  r=1e-6 Ohm  g=0 1/Ohm  i_specify=off  i_priority=None  i=0 A  i_nominal_specify=off  i_nominal_value=1  i_nominal_unit=A  v_specify=off  v_priority=None  v=6560*.5 V  v_nominal_specify=off  v_nominal_value=1  v_nominal_unit=V  vc_specify=on  vc_priority=None  vc=PVInverter.Vdc V  vc_nominal_specify=off  vc_nominal_value=1  vc_nominal_unit=V
  Constant : Constant  Value=PVInverter.Vdc
  ERef1 : fl_lib/Electrical/Electrical Elements/Electrical Reference
  PS-Simulink Converter : nesl_utility/PS-Simulink Converter  PhysicalDomain=network_engine_domain  SubClassName=ps_output  LeftPortType=input  RightPortType=output  PseudoPeriodic=off  Frequencies=[]  VectorFormat=inherit  Unit=inherit  AffineConversion=off
  Simulink-PS Converter2 : nesl_utility/Simulink-PS Converter  PhysicalDomain=network_engine_domain  SubClassName=ps_input  LeftPortType=input  RightPortType=output  PseudoPeriodic=off  Frequencies=[]  NoiseDistribution=none  NoiseParameters=[]  Unit=1  AffineConversion=off  FilteringAndDerivatives=provide  SimscapeFilterOrder=1  InputFilterTimeConstant=0.001  UdotUserProvided=0
  Simulink-PS Converter3 : nesl_utility/Simulink-PS Converter  PhysicalDomain=network_engine_domain  SubClassName=ps_input  LeftPortType=input  RightPortType=output  PseudoPeriodic=off  Frequencies=[]  NoiseDistribution=none  NoiseParameters=[]  Unit=1  AffineConversion=off  FilteringAndDerivatives=provide  SimscapeFilterOrder=1  InputFilterTimeConstant=0.001  UdotUserProvided=0
  Unit Delay : UnitDelay  SampleTime=-1  HasFrameUpgradeWarning=on
  Voltage Sensor : fl_lib/Electrical/Electrical Sensors/Voltage Sensor
  battery : batteryecm_lib/Battery  Vnom=battery.vbat_nominal V  prm_dir=simscape.enum.battery.prm_dir.disabled  R1_dis=2 Ohm  R1_ch=2 Ohm  R1=battery.resistance Ohm  prm_AH=simscape.enum.battery.prm_AH.finite  AH=battery.capacity A*hr  V1=battery.vbat_1 V  AH1=battery.charge_vbat1 A*hr  prm_R2=simscape.enum.battery.prm_R2.disabled  R2=2000 Ohm  Tmeas=298.15 K  charge_measurement_port=simscape.enum.battery.enable.no  prm_dyn=simscape.enum.battery.prm_dyn.off  Rp1=0.005 Ohm  tau1=30 s  Rp2=0.005 Ohm  tau2=30 s  Rp3=0.005 Ohm  tau3=30 s  Rp4=0.005 Ohm  tau4=30 s  Rp5=0.005 Ohm  tau5=30 s  prm_fade=simscape.enum.battery.prm_fade.disabled  N_fade=100  AH_fade=45 A*hr  R1_fade=2.02 Ohm  R1_ch_fade=2.02 Ohm  V1_fade=10.35 V  prm_age=simscape.enum.battery.prm_age.disabled  prm_age_OCV=simscape.enum.battery.prm_age_OCV.OCV  OCV_age=0.9  SOC_age=60  Tmeas_age=298.15 K  delta_time_age_vec=[0] d  temperature_age_vec=[273] K  OCV_scaling_age=2.2134e6  OCV_offset_age=1.632e6  temp_exp_age=0.515833569 V  t_exp_age=0.75  Vnom_T2=12 V  R1_T2=2.2 Ohm  R1_T2_dis=2.2 Ohm  R1_T2_ch=2.2 Ohm  V1_T2=11.4 V  R2_T2=2200 Ohm  Rp1_T2=0.005 Ohm  tau1_T2=30 s  Rp2_T2=0.005 Ohm  tau2_T2=30 s  Rp3_T2=0.005 Ohm  tau3_T2=30 s  Rp4_T2=0.005 Ohm  tau4_T2=30 s  Rp5_T2=0.005 Ohm  tau5_T2=30 s  Tmeas2=273.15 K  thermal_port=simscape.enum.thermaleffects.omit  thermal_mass=30000 J/K  i_specify=off  i_priority=None  i=0 A  i_nominal_specify=off  i_nominal_value=1  i_nominal_unit=A  v_specify=on  v_priority=None  v=6000 V  v_nominal_specify=off  v_nominal_value=1  v_nominal_unit=V  charge_specify=off  charge_priority=High  charge=50 A*hr  charge_nominal_specify=off  charge_nominal_value=1  charge_nominal_unit=A*hr  num_cycles_specify=off  num_cycles_priority=High  num_cycles=0  num_cycles_nominal_specify=off  num_cycles_nominal_value=1  num_cycles_nominal_unit=1  temperature_specify=off  temperature_priority=High  temperature=298.15 K  temperature_nominal_specify=off  temperature_nominal_value=1  temperature_nominal_unit=K
  abc : PMIOPort  Side=Right
  wires:
  Constant/1 -> Unit Delay/1
  Unit Delay/1 -> Simulink-PS Converter3/1
  m_abc/1 -> Simulink-PS Converter2/1
  PS-Simulink Converter/1 -> [Vdc]
  connections:
  Average-Value DC-DC Converter/RConn2 -- Voltage Sensor/RConn2 -- Capacitor/RConn1 -- Average-Value Voltage Source Converter (Three-Phase)/RConn2 -- ERef1/LConn1
  Average-Value DC-DC Converter/RConn1 -- Capacitor/LConn1 -- Average-Value Voltage Source Converter (Three-Phase)/RConn1 -- Voltage Sensor/LConn1
  Simulink-PS Converter3/RConn1 -- Average-Value DC-DC Converter/LConn1
  Average-Value Voltage Source Converter (Three-Phase)/LConn1 -- Simulink-PS Converter2/RConn1
  battery/RConn1 -- Average-Value DC-DC Converter/LConn3
  battery/LConn1 -- Average-Value DC-DC Converter/LConn2
  PS-Simulink Converter/LConn1 -- Voltage Sensor/RConn1
  abc/RConn1 -- Average-Value Voltage Source Converter (Three-Phase)/LConn2

== system AdmittanceScanPRBS/Renewable Plant/PV Plant/60 MWhr Battery Energy Storage/Measurement5 ==
  In1 : Inport
  u : Inport  Port=2
  Gain : Gain  Gain=sqrt((2/3))*Base.KV_base_new
  Gain1 : Gain  Gain=sqrt((1/3))*(Base.MVA_base_new/Base.KV_base_new)
  Lead-Lag (Discrete or Continuous) : eeGeneralControl/Lead-Lag (Discrete or Continuous)  T1=0  T2=PVController.t_sensor  B=inf  A=-inf  init_option=Inherited from block input  x0=0  Ts=Ts
      settings: LibrarySourceBlock=|
      | ee_sl_lib/General Control/Lead-Lag
      | (Discrete or Continuous)
  Lead-Lag (Discrete or Continuous)1 : eeGeneralControl/Lead-Lag (Discrete or Continuous)  T1=0  T2=PVController.t_sensor  B=inf  A=-inf  init_option=Inherited from block input  x0=0  Ts=Ts
      settings: LibrarySourceBlock=|
      | ee_sl_lib/General Control/Lead-Lag
      | (Discrete or Continuous)
  Out Bus Element : Outport  PortName=ipv1  Element=1
  Out Bus Element1 : Outport  Port=2  PortName=Bat  Element=Vabc_bat
  Out Bus Element2 : Outport  Port=2  PortName=Bat  Element=Iabc_bat
  wires:
  u/1 -> Lead-Lag (Discrete or Continuous)1/1
  Lead-Lag (Discrete or Continuous)1/1 -> Gain1/1, Out Bus Element/1
  In1/1 -> Lead-Lag (Discrete or Continuous)/1
  Lead-Lag (Discrete or Continuous)/1 -> Gain/1
  Gain/1 -> Out Bus Element1/1
  Gain1/1 -> Out Bus Element2/1

== system AdmittanceScanPRBS/Renewable Plant/PV Plant/60 MWhr Battery Energy Storage/Variant Subsystem ==
  ipv2 : Inport
  Vbus : Inport  Port=2
  LVRT_iq : Inport  Port=3
  Bat : Inport  Port=4
  Grid Following Support : Subsystem  VariantControl=BESSGridSupporting
      mask Display: image('$imagefile'); % Use "Edit Image" on toolstrip to change.
  Grid Forming VSM : Subsystem  VariantControl=BESSVSMControl
      mask Display: image('$imagefile'); % Use "Edit Image" on toolstrip to change.
  mabc : Outport

== system AdmittanceScanPRBS/Renewable Plant/PV Plant/PV Plant Controller /Voltage VAR Control & LVRT, FRT ==
  In Bus Element : Inport  PortName=Vbus  Element=Vmag
  In Bus Element1 : Inport  PortName=Vbus  Element=w
  Data Type Conversion : DataTypeConversion  Commented=on  RndMeth=Nearest  SaturateOnIntegerOverflow=off
  Frequency RideThrough : Subsystem  Commented=on
  LVRT Characterstics : Subsystem  Commented=on
  OR : Logic  Operator=OR  IconShape=distinctive  AllPortsSameDT=off  OutDataTypeStr=boolean
  Unit Delay : UnitDelay  Commented=on  SampleTime=-1  HasFrameUpgradeWarning=on
  V_ref : Constant  Value=PVController.V_ref  SampleTime=Ts
  Voltage Control : Subsystem
  Out Bus Element : Outport  PortName=LVRT  Element=breaker
  Out Bus Element1 : Outport  PortName=LVRT  Element=iq
  Q_ref : Outport  Port=2
  wires:
  In Bus Element/1 -> LVRT Characterstics/1(Vmag), Voltage Control/1(In1)
  LVRT Characterstics/2(iq) -> Out Bus Element1/1
  V_ref/1 -> Voltage Control/2(In2)
  Voltage Control/1(Out1) -> Q_ref/1
  OR/1 -> Data Type Conversion/1
  LVRT Characterstics/1(Trip Signal) -> OR/1
  In Bus Element1/1 -> Frequency RideThrough/1(f)
  Data Type Conversion/1 -> Unit Delay/1
  Frequency RideThrough/1(Trip  Signal) -> OR/2
  Unit Delay/1 -> Out Bus Element/1

== system AdmittanceScanPRBS/Renewable Plant/Wind Farm/Voltage VAR Control & LVRT, FRT/Frequency RideThrough ==
  f : Inport
  Avoid Operation : Subsystem
  Discrete-Time Integrator1 : DiscreteIntegrator  ExternalReset=either  SampleTime=Ts  ICPrevOutput=DiscIntNeverNeededParam  ICPrevScaledInput=DiscIntNeverNeededParam
  Duration of f<fth : Lookup_n-D  NumberOfTableDimensions=1  BreakpointsForDimension1=(1+[-0.021,-0.02,0.02,0.021])*grid.frequency  Table=[1,0,0,1]  InterpMethod=Flat  InternalRulePriority=Speed  RndMeth=Simplest
  Frequency vs Trip time : Lookup_n-D  NumberOfTableDimensions=1  BreakpointsForDimension1=frt.frequency  Table=frt.time  InterpMethod=Flat  InternalRulePriority=Speed  RndMeth=Simplest
  GreaterThan : RelationalOperator  Operator=>  OutDataTypeStr=boolean  RndMeth=Simplest  InputSameDT=off
  Trip  Signal : Outport
  wires:
  Discrete-Time Integrator1/1 -> GreaterThan/1
  Frequency vs Trip time/1 -> GreaterThan/2
  GreaterThan/1 -> Trip  Signal/1
  Duration of f<fth/1 -> Discrete-Time Integrator1/2, Discrete-Time Integrator1/1
  Avoid Operation/1(f) -> Duration of f<fth/1, Frequency vs Trip time/1
  f/1 -> Avoid Operation/1(f_in)

== system AdmittanceScanPRBS/Renewable Plant/Wind Farm/Voltage VAR Control & LVRT, FRT/LVRT Characterstics ==
  Vmag : Inport
  Discrete-Time Integrator1 : DiscreteIntegrator  ExternalReset=either  SampleTime=Ts  ICPrevOutput=DiscIntNeverNeededParam  ICPrevScaledInput=DiscIntNeverNeededParam
  Duration of Vmag<Vth : Lookup_n-D  NumberOfTableDimensions=1  BreakpointsForDimension1=[0,.9,0.91,1.2]  Table=[1,1,0,0]  InterpMethod=Flat  InternalRulePriority=Speed  RndMeth=Simplest
  Gain1 : Gain  Gain=-1
  GreaterThan : RelationalOperator  Operator=>  OutDataTypeStr=boolean  RndMeth=Simplest  InputSameDT=off
  Saturation2 : Saturate  UpperLimit=1/8  LowerLimit=-1
  Vmag vs Trip time : Lookup_n-D  NumberOfTableDimensions=1  BreakpointsForDimension1=lvrt.voltage  Table=lvrt.time  InterpMethod=Flat  InternalRulePriority=Speed  RndMeth=Simplest
  Vmag vs iq : Lookup_n-D  NumberOfTableDimensions=1  BreakpointsForDimension1=lvrt.voltageiq  Table=lvrt.iq  InternalRulePriority=Speed  RndMeth=Simplest
  Trip Signal : Outport
  iq : Outport  Port=2
  wires:
  Duration of Vmag<Vth/1 -> Discrete-Time Integrator1/2, Discrete-Time Integrator1/1
  GreaterThan/1 -> Trip Signal/1
  Discrete-Time Integrator1/1 -> GreaterThan/1
  Vmag vs Trip time/1 -> GreaterThan/2
  Vmag vs iq/1 -> Saturation2/1
  Gain1/1 -> iq/1
  Saturation2/1 -> Gain1/1
  Vmag/1 -> Vmag vs iq/1, Vmag vs Trip time/1, Duration of Vmag<Vth/1

== system AdmittanceScanPRBS/Renewable Plant/Wind Farm/Voltage VAR Control & LVRT, FRT/Voltage Control ==
  In1 : Inport
  In2 : Inport  Port=2
  Constant2 : Constant  Value=0
  Gain : Gain  Gain=windController.mv
  Sum2 : Sum  Inputs=|+-
  Switch1 : Switch  Threshold=.9  SaturateOnIntegerOverflow=off  InputSameDT=off
  Out1 : Outport
  wires:
  Gain/1 -> Out1/1
  Sum2/1 -> Switch1/1
  Switch1/1 -> Gain/1
  In1/1 -> Sum2/2, Switch1/2
  Constant2/1 -> Switch1/3
  In2/1 -> Sum2/1

== system AdmittanceScanPRBS/Renewable Plant/PV Plant/60 MWhr Battery Energy Storage/Variant Subsystem/Grid Following Support ==
  In Bus Element : Inport  PortName=Vbus
  In Bus Element1 : Inport  Port=2  PortName=ipv2
  LVRT_iq : Inport  Port=3
  GFL Battery Controller : Subsystem  mask{Vref=GFLBatteryController.V_ref, fref=GFLBatteryController.f_ref, Pref=GFLBatteryController.P_ref, Qref=GFLBatteryController.Q_ref, mp=GFLBatteryController.m_p, mv=GFLBatteryController.m_v, P=Real power, MVA=Base.MVA_base_new, zbase=Base.MVA_base_new, L=PVInverter.L, Imax=PVInverter.I_max_pu, Td=GFLBatteryController.Td, Kpic=PVController.Kp_ic, Kiic=PVController.Ki_ic, Kd=PVController.Kd}
      mask prompts: Vref "Voltage reference (PU)"; fref "Frequency reference (Hz)"; Pref "Real power reference (PU)"; Qref "Reactive power reference (PU)"; mp "Real power droop cofficient"; mv "Reactive power droop cofficient"; P "Priority mode"; MVA "Base Power (V*A)"; zbase "Base Impedance (Ohm)"; L "Filter Inductance (H)"; Imax "Inverter current limit (pu)"; Td "Sensor time delay (s)"; Kpic "Proportional gain"; Kiic "Integral gain"; Kd "Derevative gain"
      mask TypeOptions P: Real power  | Reactive power
      mask DialogControl Container4 Prompt: General
      mask DialogControl Container5 Prompt: Current Controller
      mask Display: image('$imagefile'); % Use "Edit Image" on toolstrip to change.
  mabc : Outport
  wires:
  In Bus Element/1 -> GFL Battery Controller/1(Vbus)
  LVRT_iq/1 -> GFL Battery Controller/3(LVRT_iq)
  In Bus Element1/1 -> GFL Battery Controller/2(ipv2)
  GFL Battery Controller/1(m_abc) -> mabc/1
